simulink model "uncertainities"  (R2021a)
settings: Solver=VariableStepAuto  StartTime=0.0  StopTime=10.0  RelTol=1e-3
settings Model: Creator=jessilbijou  LastModifiedBy=jessilbijou

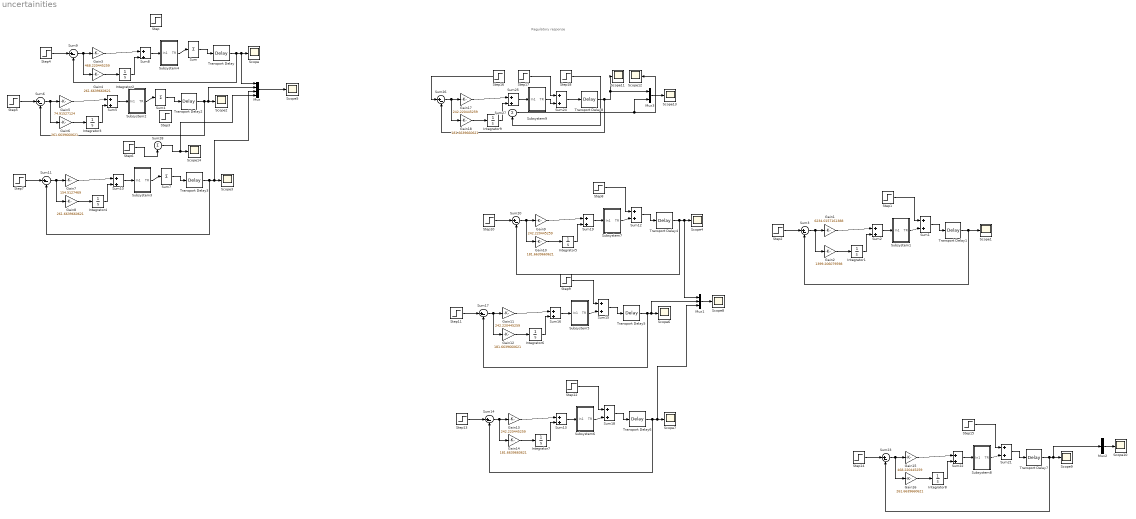
== system uncertainities ==
  note: Regulatory response
  Gain1 : Gain  Gain=6234.0157161388
  Gain{10,12,14,18} (4 alike) : Gain  Gain=181.6639660621
  Gain{9,11,13,17} (4 alike) : Gain  Gain=242.220445259
  Gain15 : Gain  Gain=468.220445259
  Gain{4,6,8,16} (4 alike) : Gain  Gain=261.6639660621
  Gain2 : Gain  Gain=1399.206079598
  Gain3 : Gain  Gain=468.220445259
  Gain5 : Gain  Gain=74.91527124
  Gain7 : Gain  Gain=154.5127469
  Integrator{1..9} (9 alike) : Integrator
  Mux : Mux
  Mux1 : Mux  Inputs=3
  Mux2 : Mux  Inputs=3
  Mux3 : Mux  Inputs=2
  Scope{,1..14} (15 alike) : Scope
  Step{,3,8..9,12} (5 alike) : Step  Time=400  After=-0.2  SampleTime=0
  Step1 : Step  Time=400  After=-0.4  SampleTime=0
  Step{10..11,13..14,18} (5 alike) : Step  Time=0  Before=415  After=418  SampleTime=0
  Step15 : Step  SampleTime=0
  Step16 : Step  Time=80  Before=415  After=418  SampleTime=0
  Step17 : Step  Time=400  After=0.2  SampleTime=0
  Step2 : Step  Time=10  Before=415  After=418  SampleTime=0
  Step{4..7} (4 alike) : Step  Time=70  Before=415  After=418  SampleTime=0
  Subsystem1 : Subsystem
  Subsystem2 : Subsystem
  Subsystem3 : Subsystem
  Subsystem4 : Subsystem
  Subsystem5 : Subsystem
  Subsystem6 : Subsystem
  Subsystem7 : Subsystem
  Subsystem8 : Subsystem
  Subsystem9 : Subsystem
  Sum{,4,7,27..28} (5 alike) : Sum  Inputs=|+
  Sum{1..2,5,8,10,12..13,15..16,18..19,21..22,24..25} (15 alike) : Sum  Inputs=|++
  Sum{3,6,9,11,14,17,20,23,26} (9 alike) : Sum  Inputs=|+-
  Transport Delay{,1..8} (9 alike) : TransportDelay  DelayTime=0
  wires:
  Gain8/1 -> Integrator4/1
  Sum8/1 -> Subsystem4/1(In1)
  Integrator3/1 -> Sum5/2
  Subsystem3/1(TR) -> Sum7/1
  Mux/1 -> Scope5/1
  Step5/1 -> Sum6/1
  Sum/1 -> Transport Delay/1
  Sum4/1 -> Transport Delay2/1
  Step7/1 -> Sum11/1
  Sum10/1 -> Subsystem3/1(In1)
  Gain4/1 -> Integrator2/1
  Transport Delay2/1 -> Sum6/2, Mux/2, Scope2/1
  Gain6/1 -> Integrator3/1
  Sum6/1 -> Gain6/1, Gain5/1
  Integrator2/1 -> Sum8/2
  Sum7/1 -> Transport Delay3/1
  Sum9/1 -> Gain4/1, Gain3/1
  Step4/1 -> Sum9/1
  Integrator4/1 -> Sum10/2
  Gain7/1 -> Sum10/1
  Transport Delay/1 -> Sum9/2, Mux/1, Scope/1
  Subsystem4/1(TR) -> Sum/1
  Sum5/1 -> Subsystem2/1(In1)
  Gain3/1 -> Sum8/1
  Subsystem2/1(TR) -> Sum4/1
  Sum11/1 -> Gain8/1, Gain7/1
  Gain5/1 -> Sum5/1
  Transport Delay3/1 -> Sum11/2, Mux/3, Scope3/1
  Step6/1 -> Sum28/1
  Sum28/1 -> Mux/4, Scope14/1
  Step17/1 -> Sum24/1
  Mux3/1 -> Scope13/1
  Sum26/1 -> Gain18/1, Gain17/1
  Step18/1 -> Sum27/1
  Transport Delay8/1 -> Sum26/2, Mux3/1, Scope11/1
  Sum24/1 -> Transport Delay8/1
  Integrator9/1 -> Sum25/2
  Gain17/1 -> Sum25/1
  Subsystem9/1(TR) -> Sum24/2
  Sum25/1 -> Subsystem9/1(In1)
  Sum27/1 -> Mux3/2, Scope12/1
  Gain18/1 -> Integrator9/1
  Step16/1 -> Sum26/1
  Sum3/1 -> Gain2/1, Gain1/1
  Gain1/1 -> Sum2/1
  Transport Delay7/1 -> Sum23/2, Mux2/2, Scope9/1
  Sum2/1 -> Subsystem1/1(In1)
  Subsystem6/1(TR) -> Sum18/2
  Subsystem1/1(TR) -> Sum1/2
  Step10/1 -> Sum20/1
  Subsystem7/1(TR) -> Sum12/2
  Sum16/1 -> Subsystem5/1(In1)
  Gain10/1 -> Integrator5/1
  Gain15/1 -> Sum22/1
  Sum1/1 -> Transport Delay1/1
  Integrator5/1 -> Sum19/2
  Step9/1 -> Sum15/1
  Step1/1 -> Sum1/1
  Subsystem5/1(TR) -> Sum15/2
  Transport Delay5/1 -> Sum17/2, Mux1/2, Scope6/1
  Step14/1 -> Sum23/1
  Sum17/1 -> Gain12/1, Gain11/1
  Sum13/1 -> Subsystem6/1(In1)
  Integrator1/1 -> Sum2/2
  Sum15/1 -> Transport Delay5/1
  Gain9/1 -> Sum19/1
  Transport Delay1/1 -> Sum3/2, Scope1/1
  Integrator6/1 -> Sum16/2
  Step12/1 -> Sum18/1
  Transport Delay6/1 -> Sum14/2, Mux1/3, Scope7/1
  Step11/1 -> Sum17/1
  Integrator7/1 -> Sum13/2
  Gain13/1 -> Sum13/1
  Sum19/1 -> Subsystem7/1(In1)
  Step15/1 -> Sum21/1
  Sum21/1 -> Transport Delay7/1
  Gain16/1 -> Integrator8/1
  Sum14/1 -> Gain14/1, Gain13/1
  Gain11/1 -> Sum16/1
  Sum22/1 -> Subsystem8/1(In1)
  Transport Delay4/1 -> Sum20/2, Mux1/1, Scope4/1
  Step8/1 -> Sum12/1
  Gain2/1 -> Integrator1/1
  Step13/1 -> Sum14/1
  Sum18/1 -> Transport Delay6/1
  Sum12/1 -> Transport Delay4/1
  Sum23/1 -> Gain16/1, Gain15/1
  Subsystem8/1(TR) -> Sum21/2
  Gain14/1 -> Integrator7/1
  Integrator8/1 -> Sum22/2
  Gain12/1 -> Integrator6/1
  Step2/1 -> Sum3/1
  Mux2/1 -> Scope10/1
  Mux1/1 -> Scope8/1
  Sum20/1 -> Gain10/1, Gain9/1

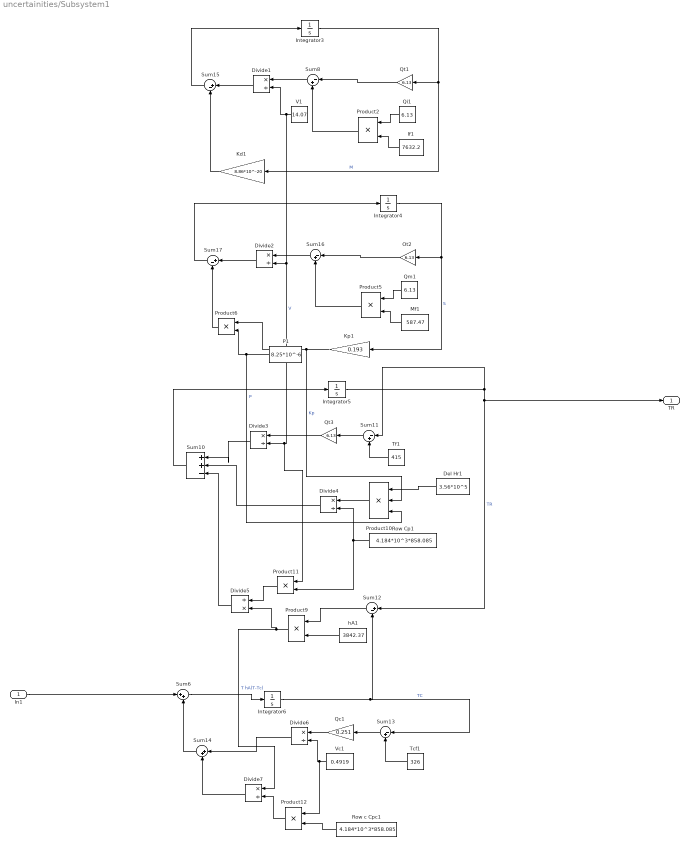
== system uncertainities/Subsystem1 ==
  In1 : Inport
  Del Hr1 : Constant  Value=3.56*10^5
  Divide{1..4,6..7} (6 alike) : Product  Inputs=*/
  Divide5 : Product  Inputs=/*
  If1 : Constant  Value=7632.2
  Integrator3 : Integrator  InitialCondition=7632.2
  Integrator4 : Integrator  InitialCondition=587.47
  Integrator5 : Integrator  InitialCondition=415
  Integrator6 : Integrator  InitialCondition=326
  Kd1 : Gain  Gain=8.86*10^-20
  Kp1 : Gain  Gain=0.193
  Mf1 : Constant  Value=587.47
  Ot2 : Gain  Gain=6.13
  P1 : Constant  Value=8.25*10^-6
  Product10 : Product  Inputs=3
  Product{2,5..6,9,11..12} (6 alike) : Product
  Qc1 : Gain  Gain=0.251
  Qi1 : Constant  Value=6.13
  Qm1 : Constant  Value=6.13
  Qt1 : Gain  Gain=6.13
  Qt3 : Gain  Gain=6.13
  Row Cp1 : Constant  Value=4.184*10^3*858.085
  Row c Cpc1 : Constant  Value=4.184*10^3*858.085
  Sum10 : Sum  Inputs=|++-
  Sum{8,11,13,16} (4 alike) : Sum  Inputs=|-+
  Sum12 : Sum  Inputs=|+-
  Sum14 : Sum  Inputs=|++
  Sum15 : Sum  Inputs=|+-
  Sum17 : Sum  Inputs=|+-
  Sum6 : Sum  Inputs=|++
  Tcf1 : Constant  Value=326
  Tf1 : Constant  Value=415
  V1 : Constant  Value=14.07
  Vc1 : Constant  Value=0.4919
  hA1 : Constant  Value=3842.37
  TR : Outport
  wires:
  Qm1/1 -> Product5/1
  Sum12/1 -> Product9/1
  Sum10/1 -> Integrator5/1
  Integrator5/1 -> TR/1, Sum12/1, Sum11/1  "TR"
  Ot2/1 -> Sum16/1
  Product11/1 -> Divide5/1
  Divide4/1 -> Sum10/2
  Sum16/1 -> Divide2/1
  Del Hr1/1 -> Product10/1
  Qi1/1 -> Product2/1
  Divide5/1 -> Sum10/3
  hA1/1 -> Product9/2
  Row c Cpc1/1 -> Product12/2
  Product10/1 -> Divide4/1
  Kd1/1 -> Sum15/2
  If1/1 -> Product2/2
  Divide3/1 -> Sum10/1
  Product6/1 -> Sum17/2
  Mf1/1 -> Product5/2
  Sum17/1 -> Integrator4/1
  Qt1/1 -> Sum8/1
  Kp1/1 -> Product6/1, Product10/2  "Kp"
  Tcf1/1 -> Sum13/2
  Integrator3/1 -> Kd1/1, Qt1/1  "M"
  Product9/1 -> Divide5/2, Divide7/1  "T hA(T-Tc)"
  Sum15/1 -> Integrator3/1
  Row Cp1/1 -> Product11/2, Divide4/2
  Sum11/1 -> Qt3/1
  Divide1/1 -> Sum15/1
  Product5/1 -> Sum16/2
  P1/1 -> Product6/2, Product10/3  "P"
  Vc1/1 -> Product12/1, Divide6/2
  Product2/1 -> Sum8/2
  V1/1 -> Product11/1, Divide3/2, Divide2/2, Divide1/2  "V"
  Sum8/1 -> Divide1/1
  Integrator4/1 -> Kp1/1, Ot2/1  "S"
  Divide6/1 -> Sum14/1
  Divide2/1 -> Sum17/1
  Divide7/1 -> Sum14/2
  Tf1/1 -> Sum11/2
  Qc1/1 -> Divide6/1
  Sum13/1 -> Qc1/1
  Product12/1 -> Divide7/2
  Integrator6/1 -> Sum13/1, Sum12/2  "TC"
  Qt3/1 -> Divide3/1
  Sum14/1 -> Sum6/2
  In1/1 -> Sum6/1
  Sum6/1 -> Integrator6/1

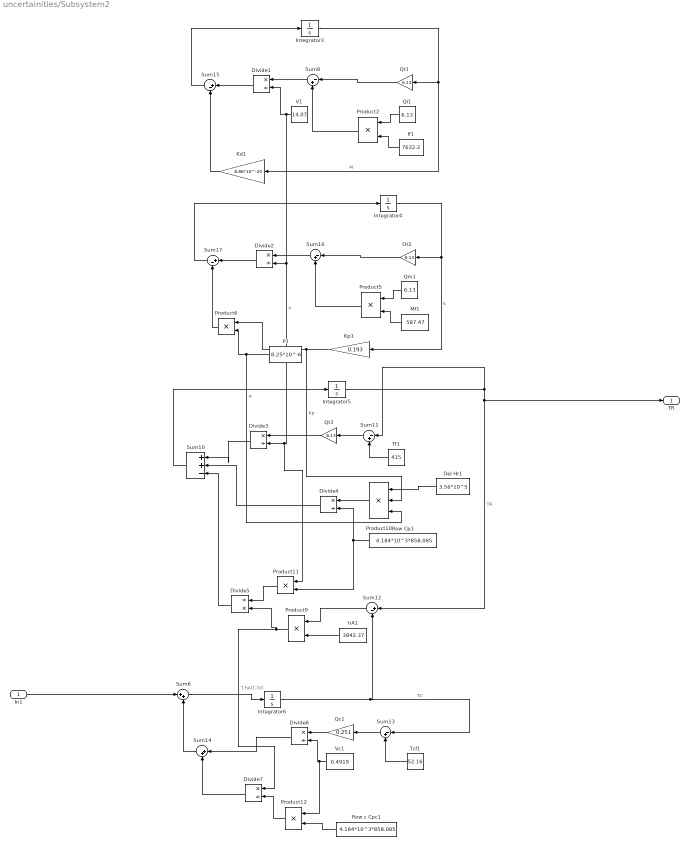
== system uncertainities/Subsystem2 ==
  In1 : Inport
  Del Hr1 : Constant  Value=3.56*10^5
  Divide{1..4,6..7} (6 alike) : Product  Inputs=*/
  Divide5 : Product  Inputs=/*
  If1 : Constant  Value=7632.2
  Integrator3 : Integrator  InitialCondition=7632.2
  Integrator4 : Integrator  InitialCondition=587.47
  Integrator5 : Integrator  InitialCondition=415
  Integrator6 : Integrator  InitialCondition=326
  Kd1 : Gain  Gain=8.86*10^-20
  Kp1 : Gain  Gain=0.193
  Mf1 : Constant  Value=587.47
  Ot2 : Gain  Gain=6.13
  P1 : Constant  Value=8.25*10^-6
  Product10 : Product  Inputs=3
  Product{2,5..6,9,11..12} (6 alike) : Product
  Qc1 : Gain  Gain=0.251
  Qi1 : Constant  Value=6.13
  Qm1 : Constant  Value=6.13
  Qt1 : Gain  Gain=6.13
  Qt3 : Gain  Gain=6.13
  Row Cp1 : Constant  Value=4.184*10^3*858.085
  Row c Cpc1 : Constant  Value=4.184*10^3*858.085
  Sum10 : Sum  Inputs=|++-
  Sum{8,11,13,16} (4 alike) : Sum  Inputs=|-+
  Sum12 : Sum  Inputs=|+-
  Sum14 : Sum  Inputs=|++
  Sum15 : Sum  Inputs=|+-
  Sum17 : Sum  Inputs=|+-
  Sum6 : Sum  Inputs=|++
  Tcf1 : Constant  Value=52.16
  Tf1 : Constant  Value=415
  V1 : Constant  Value=14.07
  Vc1 : Constant  Value=0.4919
  hA1 : Constant  Value=3842.37
  TR : Outport
  wires:
  Qm1/1 -> Product5/1
  Sum12/1 -> Product9/1
  Sum10/1 -> Integrator5/1
  Integrator5/1 -> TR/1, Sum12/1, Sum11/1  "TR"
  Ot2/1 -> Sum16/1
  Product11/1 -> Divide5/1
  Divide4/1 -> Sum10/2
  Sum16/1 -> Divide2/1
  Del Hr1/1 -> Product10/1
  Qi1/1 -> Product2/1
  Divide5/1 -> Sum10/3
  hA1/1 -> Product9/2
  Row c Cpc1/1 -> Product12/2
  Product10/1 -> Divide4/1
  Kd1/1 -> Sum15/2
  If1/1 -> Product2/2
  Divide3/1 -> Sum10/1
  Product6/1 -> Sum17/2
  Mf1/1 -> Product5/2
  Sum17/1 -> Integrator4/1
  Qt1/1 -> Sum8/1
  Kp1/1 -> Product6/1, Product10/2  "Kp"
  Tcf1/1 -> Sum13/2
  Integrator3/1 -> Kd1/1, Qt1/1  "M"
  Product9/1 -> Divide5/2, Divide7/1  "T hA(T-Tc)"
  Sum15/1 -> Integrator3/1
  Row Cp1/1 -> Product11/2, Divide4/2
  Sum11/1 -> Qt3/1
  Divide1/1 -> Sum15/1
  Product5/1 -> Sum16/2
  P1/1 -> Product6/2, Product10/3  "P"
  Vc1/1 -> Product12/1, Divide6/2
  Product2/1 -> Sum8/2
  V1/1 -> Product11/1, Divide3/2, Divide2/2, Divide1/2  "V"
  Sum8/1 -> Divide1/1
  Integrator4/1 -> Kp1/1, Ot2/1  "S"
  Divide6/1 -> Sum14/1
  Divide2/1 -> Sum17/1
  Divide7/1 -> Sum14/2
  Tf1/1 -> Sum11/2
  Qc1/1 -> Divide6/1
  Sum13/1 -> Qc1/1
  Product12/1 -> Divide7/2
  Integrator6/1 -> Sum13/1, Sum12/2  "TC"
  Qt3/1 -> Divide3/1
  Sum14/1 -> Sum6/2
  In1/1 -> Sum6/1
  Sum6/1 -> Integrator6/1

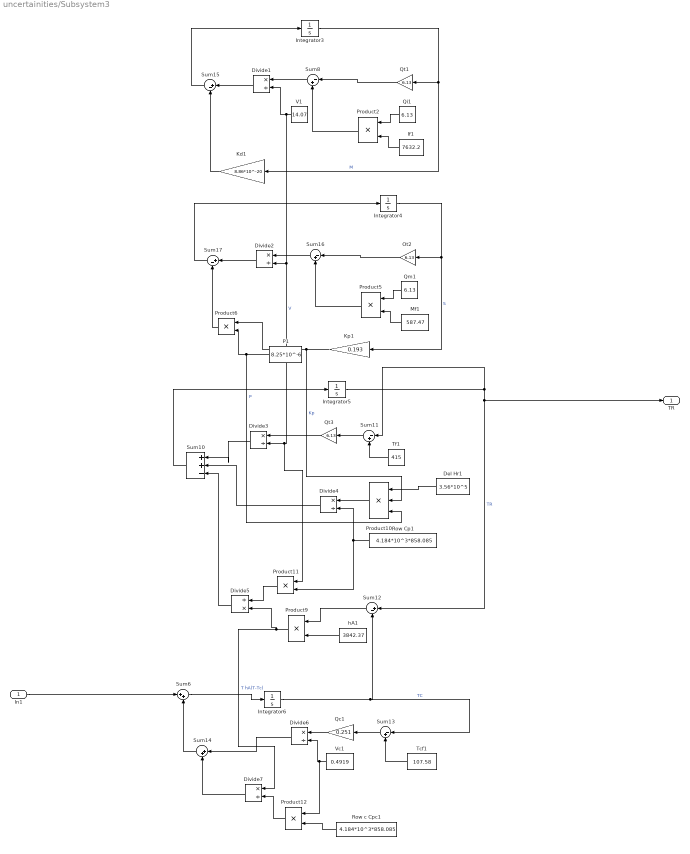
== system uncertainities/Subsystem3 ==
  In1 : Inport
  Del Hr1 : Constant  Value=3.56*10^5
  Divide{1..4,6..7} (6 alike) : Product  Inputs=*/
  Divide5 : Product  Inputs=/*
  If1 : Constant  Value=7632.2
  Integrator3 : Integrator  InitialCondition=7632.2
  Integrator4 : Integrator  InitialCondition=587.47
  Integrator5 : Integrator  InitialCondition=415
  Integrator6 : Integrator  InitialCondition=326
  Kd1 : Gain  Gain=8.86*10^-20
  Kp1 : Gain  Gain=0.193
  Mf1 : Constant  Value=587.47
  Ot2 : Gain  Gain=6.13
  P1 : Constant  Value=8.25*10^-6
  Product10 : Product  Inputs=3
  Product{2,5..6,9,11..12} (6 alike) : Product
  Qc1 : Gain  Gain=0.251
  Qi1 : Constant  Value=6.13
  Qm1 : Constant  Value=6.13
  Qt1 : Gain  Gain=6.13
  Qt3 : Gain  Gain=6.13
  Row Cp1 : Constant  Value=4.184*10^3*858.085
  Row c Cpc1 : Constant  Value=4.184*10^3*858.085
  Sum10 : Sum  Inputs=|++-
  Sum{8,11,13,16} (4 alike) : Sum  Inputs=|-+
  Sum12 : Sum  Inputs=|+-
  Sum14 : Sum  Inputs=|++
  Sum15 : Sum  Inputs=|+-
  Sum17 : Sum  Inputs=|+-
  Sum6 : Sum  Inputs=|++
  Tcf1 : Constant  Value=107.58
  Tf1 : Constant  Value=415
  V1 : Constant  Value=14.07
  Vc1 : Constant  Value=0.4919
  hA1 : Constant  Value=3842.37
  TR : Outport
  wires:
  Qm1/1 -> Product5/1
  Sum12/1 -> Product9/1
  Sum10/1 -> Integrator5/1
  Integrator5/1 -> TR/1, Sum12/1, Sum11/1  "TR"
  Ot2/1 -> Sum16/1
  Product11/1 -> Divide5/1
  Divide4/1 -> Sum10/2
  Sum16/1 -> Divide2/1
  Del Hr1/1 -> Product10/1
  Qi1/1 -> Product2/1
  Divide5/1 -> Sum10/3
  hA1/1 -> Product9/2
  Row c Cpc1/1 -> Product12/2
  Product10/1 -> Divide4/1
  Kd1/1 -> Sum15/2
  If1/1 -> Product2/2
  Divide3/1 -> Sum10/1
  Product6/1 -> Sum17/2
  Mf1/1 -> Product5/2
  Sum17/1 -> Integrator4/1
  Qt1/1 -> Sum8/1
  Kp1/1 -> Product6/1, Product10/2  "Kp"
  Tcf1/1 -> Sum13/2
  Integrator3/1 -> Kd1/1, Qt1/1  "M"
  Product9/1 -> Divide5/2, Divide7/1  "T hA(T-Tc)"
  Sum15/1 -> Integrator3/1
  Row Cp1/1 -> Product11/2, Divide4/2
  Sum11/1 -> Qt3/1
  Divide1/1 -> Sum15/1
  Product5/1 -> Sum16/2
  P1/1 -> Product6/2, Product10/3  "P"
  Vc1/1 -> Product12/1, Divide6/2
  Product2/1 -> Sum8/2
  V1/1 -> Product11/1, Divide3/2, Divide2/2, Divide1/2  "V"
  Sum8/1 -> Divide1/1
  Integrator4/1 -> Kp1/1, Ot2/1  "S"
  Divide6/1 -> Sum14/1
  Divide2/1 -> Sum17/1
  Divide7/1 -> Sum14/2
  Tf1/1 -> Sum11/2
  Qc1/1 -> Divide6/1
  Sum13/1 -> Qc1/1
  Product12/1 -> Divide7/2
  Integrator6/1 -> Sum13/1, Sum12/2  "TC"
  Qt3/1 -> Divide3/1
  Sum14/1 -> Sum6/2
  In1/1 -> Sum6/1
  Sum6/1 -> Integrator6/1

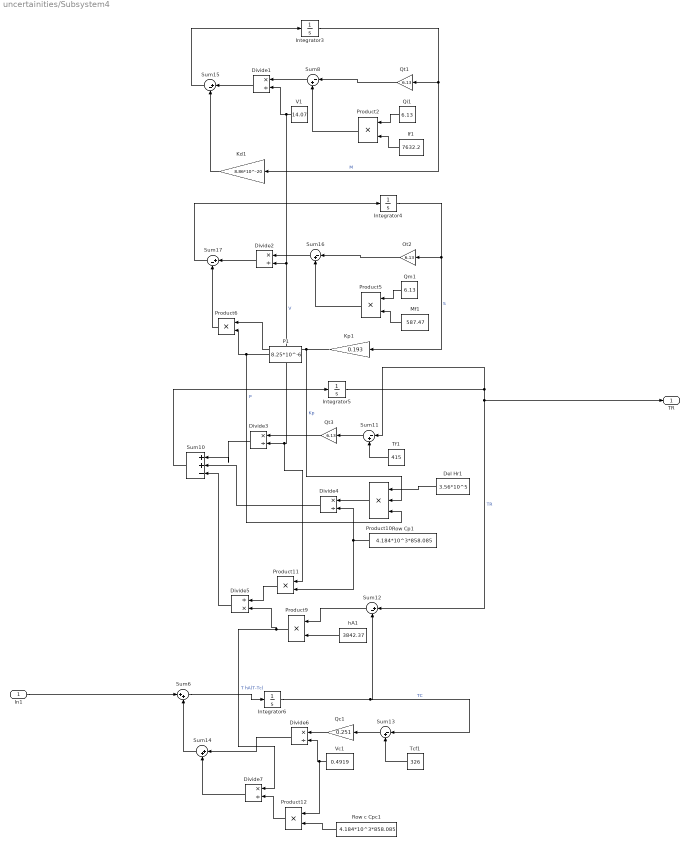
== system uncertainities/Subsystem4 ==
  In1 : Inport
  Del Hr1 : Constant  Value=3.56*10^5
  Divide{1..4,6..7} (6 alike) : Product  Inputs=*/
  Divide5 : Product  Inputs=/*
  If1 : Constant  Value=7632.2
  Integrator3 : Integrator  InitialCondition=7632.2
  Integrator4 : Integrator  InitialCondition=587.47
  Integrator5 : Integrator  InitialCondition=415
  Integrator6 : Integrator  InitialCondition=326
  Kd1 : Gain  Gain=8.86*10^-20
  Kp1 : Gain  Gain=0.193
  Mf1 : Constant  Value=587.47
  Ot2 : Gain  Gain=6.13
  P1 : Constant  Value=8.25*10^-6
  Product10 : Product  Inputs=3
  Product{2,5..6,9,11..12} (6 alike) : Product
  Qc1 : Gain  Gain=0.251
  Qi1 : Constant  Value=6.13
  Qm1 : Constant  Value=6.13
  Qt1 : Gain  Gain=6.13
  Qt3 : Gain  Gain=6.13
  Row Cp1 : Constant  Value=4.184*10^3*858.085
  Row c Cpc1 : Constant  Value=4.184*10^3*858.085
  Sum10 : Sum  Inputs=|++-
  Sum{8,11,13,16} (4 alike) : Sum  Inputs=|-+
  Sum12 : Sum  Inputs=|+-
  Sum14 : Sum  Inputs=|++
  Sum15 : Sum  Inputs=|+-
  Sum17 : Sum  Inputs=|+-
  Sum6 : Sum  Inputs=|++
  Tcf1 : Constant  Value=326
  Tf1 : Constant  Value=415
  V1 : Constant  Value=14.07
  Vc1 : Constant  Value=0.4919
  hA1 : Constant  Value=3842.37
  TR : Outport
  wires:
  Qm1/1 -> Product5/1
  Sum12/1 -> Product9/1
  Sum10/1 -> Integrator5/1
  Integrator5/1 -> TR/1, Sum12/1, Sum11/1  "TR"
  Ot2/1 -> Sum16/1
  Product11/1 -> Divide5/1
  Divide4/1 -> Sum10/2
  Sum16/1 -> Divide2/1
  Del Hr1/1 -> Product10/1
  Qi1/1 -> Product2/1
  Divide5/1 -> Sum10/3
  hA1/1 -> Product9/2
  Row c Cpc1/1 -> Product12/2
  Product10/1 -> Divide4/1
  Kd1/1 -> Sum15/2
  If1/1 -> Product2/2
  Divide3/1 -> Sum10/1
  Product6/1 -> Sum17/2
  Mf1/1 -> Product5/2
  Sum17/1 -> Integrator4/1
  Qt1/1 -> Sum8/1
  Kp1/1 -> Product6/1, Product10/2  "Kp"
  Tcf1/1 -> Sum13/2
  Integrator3/1 -> Kd1/1, Qt1/1  "M"
  Product9/1 -> Divide5/2, Divide7/1  "T hA(T-Tc)"
  Sum15/1 -> Integrator3/1
  Row Cp1/1 -> Product11/2, Divide4/2
  Sum11/1 -> Qt3/1
  Divide1/1 -> Sum15/1
  Product5/1 -> Sum16/2
  P1/1 -> Product6/2, Product10/3  "P"
  Vc1/1 -> Product12/1, Divide6/2
  Product2/1 -> Sum8/2
  V1/1 -> Product11/1, Divide3/2, Divide2/2, Divide1/2  "V"
  Sum8/1 -> Divide1/1
  Integrator4/1 -> Kp1/1, Ot2/1  "S"
  Divide6/1 -> Sum14/1
  Divide2/1 -> Sum17/1
  Divide7/1 -> Sum14/2
  Tf1/1 -> Sum11/2
  Qc1/1 -> Divide6/1
  Sum13/1 -> Qc1/1
  Product12/1 -> Divide7/2
  Integrator6/1 -> Sum13/1, Sum12/2  "TC"
  Qt3/1 -> Divide3/1
  Sum14/1 -> Sum6/2
  In1/1 -> Sum6/1
  Sum6/1 -> Integrator6/1

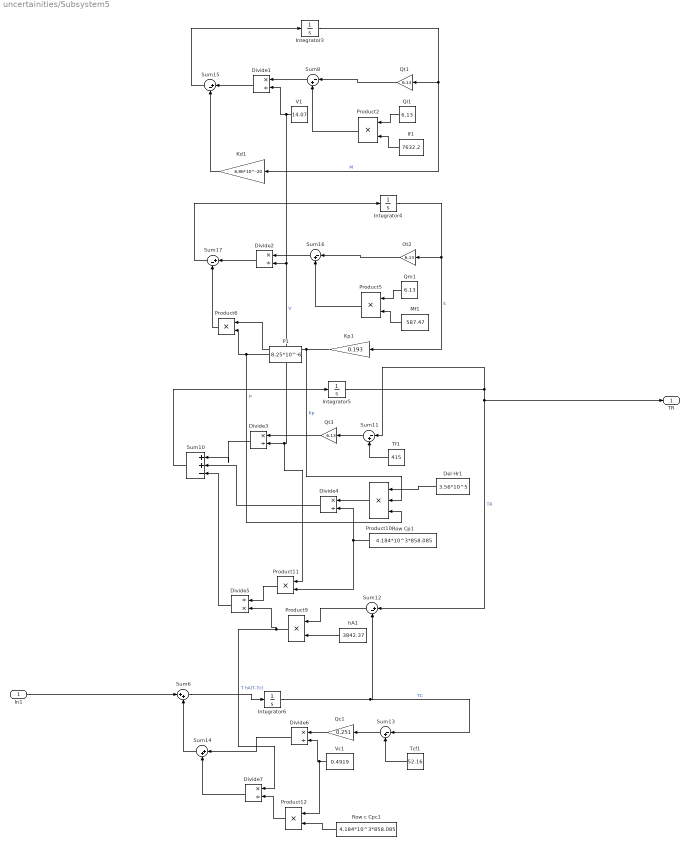
== system uncertainities/Subsystem5 ==
  In1 : Inport
  Del Hr1 : Constant  Value=3.56*10^5
  Divide{1..4,6..7} (6 alike) : Product  Inputs=*/
  Divide5 : Product  Inputs=/*
  If1 : Constant  Value=7632.2
  Integrator3 : Integrator  InitialCondition=7632.2
  Integrator4 : Integrator  InitialCondition=587.47
  Integrator5 : Integrator  InitialCondition=415
  Integrator6 : Integrator  InitialCondition=326
  Kd1 : Gain  Gain=8.86*10^-20
  Kp1 : Gain  Gain=0.193
  Mf1 : Constant  Value=587.47
  Ot2 : Gain  Gain=6.13
  P1 : Constant  Value=8.25*10^-6
  Product10 : Product  Inputs=3
  Product{2,5..6,9,11..12} (6 alike) : Product
  Qc1 : Gain  Gain=0.251
  Qi1 : Constant  Value=6.13
  Qm1 : Constant  Value=6.13
  Qt1 : Gain  Gain=6.13
  Qt3 : Gain  Gain=6.13
  Row Cp1 : Constant  Value=4.184*10^3*858.085
  Row c Cpc1 : Constant  Value=4.184*10^3*858.085
  Sum10 : Sum  Inputs=|++-
  Sum{8,11,13,16} (4 alike) : Sum  Inputs=|-+
  Sum12 : Sum  Inputs=|+-
  Sum14 : Sum  Inputs=|++
  Sum15 : Sum  Inputs=|+-
  Sum17 : Sum  Inputs=|+-
  Sum6 : Sum  Inputs=|++
  Tcf1 : Constant  Value=52.16
  Tf1 : Constant  Value=415
  V1 : Constant  Value=14.07
  Vc1 : Constant  Value=0.4919
  hA1 : Constant  Value=3842.37
  TR : Outport
  wires:
  Qm1/1 -> Product5/1
  Sum12/1 -> Product9/1
  Sum10/1 -> Integrator5/1
  Integrator5/1 -> TR/1, Sum12/1, Sum11/1  "TR"
  Ot2/1 -> Sum16/1
  Product11/1 -> Divide5/1
  Divide4/1 -> Sum10/2
  Sum16/1 -> Divide2/1
  Del Hr1/1 -> Product10/1
  Qi1/1 -> Product2/1
  Divide5/1 -> Sum10/3
  hA1/1 -> Product9/2
  Row c Cpc1/1 -> Product12/2
  Product10/1 -> Divide4/1
  Kd1/1 -> Sum15/2
  If1/1 -> Product2/2
  Divide3/1 -> Sum10/1
  Product6/1 -> Sum17/2
  Mf1/1 -> Product5/2
  Sum17/1 -> Integrator4/1
  Qt1/1 -> Sum8/1
  Kp1/1 -> Product6/1, Product10/2  "Kp"
  Tcf1/1 -> Sum13/2
  Integrator3/1 -> Kd1/1, Qt1/1  "M"
  Product9/1 -> Divide5/2, Divide7/1  "T hA(T-Tc)"
  Sum15/1 -> Integrator3/1
  Row Cp1/1 -> Product11/2, Divide4/2
  Sum11/1 -> Qt3/1
  Divide1/1 -> Sum15/1
  Product5/1 -> Sum16/2
  P1/1 -> Product6/2, Product10/3  "P"
  Vc1/1 -> Product12/1, Divide6/2
  Product2/1 -> Sum8/2
  V1/1 -> Product11/1, Divide3/2, Divide2/2, Divide1/2  "V"
  Sum8/1 -> Divide1/1
  Integrator4/1 -> Kp1/1, Ot2/1  "S"
  Divide6/1 -> Sum14/1
  Divide2/1 -> Sum17/1
  Divide7/1 -> Sum14/2
  Tf1/1 -> Sum11/2
  Qc1/1 -> Divide6/1
  Sum13/1 -> Qc1/1
  Product12/1 -> Divide7/2
  Integrator6/1 -> Sum13/1, Sum12/2  "TC"
  Qt3/1 -> Divide3/1
  Sum14/1 -> Sum6/2
  In1/1 -> Sum6/1
  Sum6/1 -> Integrator6/1

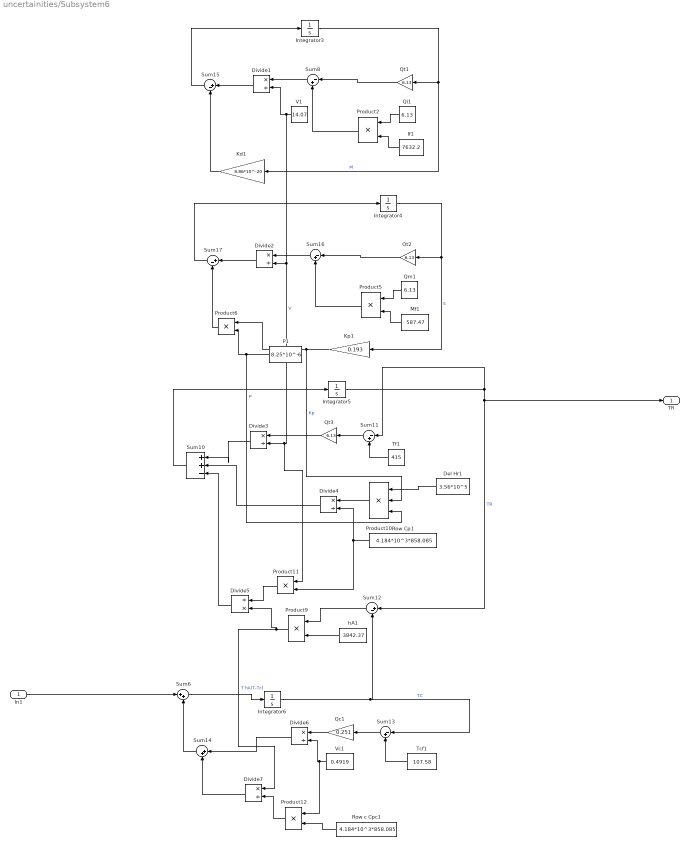
== system uncertainities/Subsystem6 ==
  In1 : Inport
  Del Hr1 : Constant  Value=3.56*10^5
  Divide{1..4,6..7} (6 alike) : Product  Inputs=*/
  Divide5 : Product  Inputs=/*
  If1 : Constant  Value=7632.2
  Integrator3 : Integrator  InitialCondition=7632.2
  Integrator4 : Integrator  InitialCondition=587.47
  Integrator5 : Integrator  InitialCondition=415
  Integrator6 : Integrator  InitialCondition=326
  Kd1 : Gain  Gain=8.86*10^-20
  Kp1 : Gain  Gain=0.193
  Mf1 : Constant  Value=587.47
  Ot2 : Gain  Gain=6.13
  P1 : Constant  Value=8.25*10^-6
  Product10 : Product  Inputs=3
  Product{2,5..6,9,11..12} (6 alike) : Product
  Qc1 : Gain  Gain=0.251
  Qi1 : Constant  Value=6.13
  Qm1 : Constant  Value=6.13
  Qt1 : Gain  Gain=6.13
  Qt3 : Gain  Gain=6.13
  Row Cp1 : Constant  Value=4.184*10^3*858.085
  Row c Cpc1 : Constant  Value=4.184*10^3*858.085
  Sum10 : Sum  Inputs=|++-
  Sum{8,11,13,16} (4 alike) : Sum  Inputs=|-+
  Sum12 : Sum  Inputs=|+-
  Sum14 : Sum  Inputs=|++
  Sum15 : Sum  Inputs=|+-
  Sum17 : Sum  Inputs=|+-
  Sum6 : Sum  Inputs=|++
  Tcf1 : Constant  Value=107.58
  Tf1 : Constant  Value=415
  V1 : Constant  Value=14.07
  Vc1 : Constant  Value=0.4919
  hA1 : Constant  Value=3842.37
  TR : Outport
  wires:
  Qm1/1 -> Product5/1
  Sum12/1 -> Product9/1
  Sum10/1 -> Integrator5/1
  Integrator5/1 -> TR/1, Sum12/1, Sum11/1  "TR"
  Ot2/1 -> Sum16/1
  Product11/1 -> Divide5/1
  Divide4/1 -> Sum10/2
  Sum16/1 -> Divide2/1
  Del Hr1/1 -> Product10/1
  Qi1/1 -> Product2/1
  Divide5/1 -> Sum10/3
  hA1/1 -> Product9/2
  Row c Cpc1/1 -> Product12/2
  Product10/1 -> Divide4/1
  Kd1/1 -> Sum15/2
  If1/1 -> Product2/2
  Divide3/1 -> Sum10/1
  Product6/1 -> Sum17/2
  Mf1/1 -> Product5/2
  Sum17/1 -> Integrator4/1
  Qt1/1 -> Sum8/1
  Kp1/1 -> Product6/1, Product10/2  "Kp"
  Tcf1/1 -> Sum13/2
  Integrator3/1 -> Kd1/1, Qt1/1  "M"
  Product9/1 -> Divide5/2, Divide7/1  "T hA(T-Tc)"
  Sum15/1 -> Integrator3/1
  Row Cp1/1 -> Product11/2, Divide4/2
  Sum11/1 -> Qt3/1
  Divide1/1 -> Sum15/1
  Product5/1 -> Sum16/2
  P1/1 -> Product6/2, Product10/3  "P"
  Vc1/1 -> Product12/1, Divide6/2
  Product2/1 -> Sum8/2
  V1/1 -> Product11/1, Divide3/2, Divide2/2, Divide1/2  "V"
  Sum8/1 -> Divide1/1
  Integrator4/1 -> Kp1/1, Ot2/1  "S"
  Divide6/1 -> Sum14/1
  Divide2/1 -> Sum17/1
  Divide7/1 -> Sum14/2
  Tf1/1 -> Sum11/2
  Qc1/1 -> Divide6/1
  Sum13/1 -> Qc1/1
  Product12/1 -> Divide7/2
  Integrator6/1 -> Sum13/1, Sum12/2  "TC"
  Qt3/1 -> Divide3/1
  Sum14/1 -> Sum6/2
  In1/1 -> Sum6/1
  Sum6/1 -> Integrator6/1

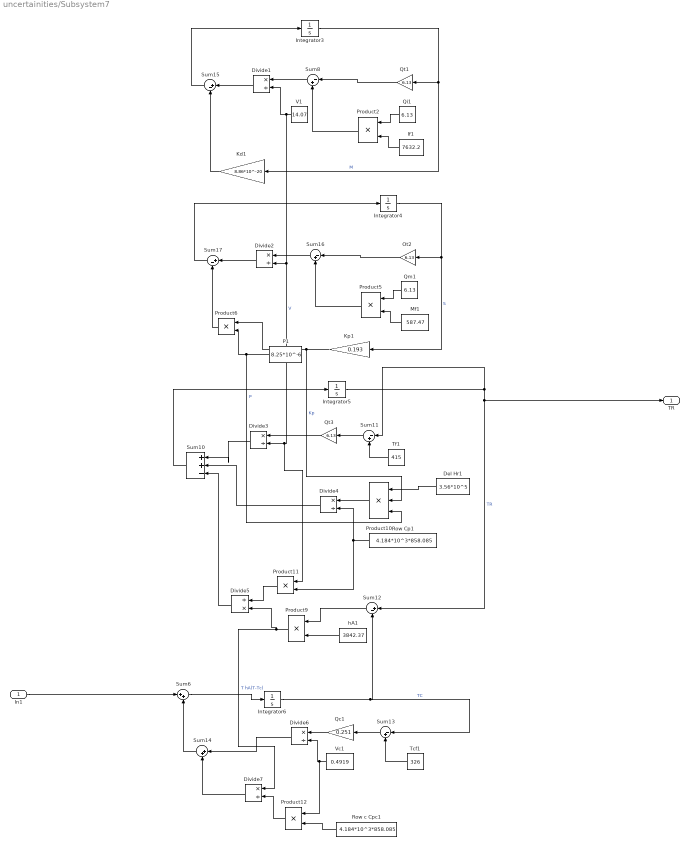
== system uncertainities/Subsystem7 ==
  In1 : Inport
  Del Hr1 : Constant  Value=3.56*10^5
  Divide{1..4,6..7} (6 alike) : Product  Inputs=*/
  Divide5 : Product  Inputs=/*
  If1 : Constant  Value=7632.2
  Integrator3 : Integrator  InitialCondition=7632.2
  Integrator4 : Integrator  InitialCondition=587.47
  Integrator5 : Integrator  InitialCondition=415
  Integrator6 : Integrator  InitialCondition=326
  Kd1 : Gain  Gain=8.86*10^-20
  Kp1 : Gain  Gain=0.193
  Mf1 : Constant  Value=587.47
  Ot2 : Gain  Gain=6.13
  P1 : Constant  Value=8.25*10^-6
  Product10 : Product  Inputs=3
  Product{2,5..6,9,11..12} (6 alike) : Product
  Qc1 : Gain  Gain=0.251
  Qi1 : Constant  Value=6.13
  Qm1 : Constant  Value=6.13
  Qt1 : Gain  Gain=6.13
  Qt3 : Gain  Gain=6.13
  Row Cp1 : Constant  Value=4.184*10^3*858.085
  Row c Cpc1 : Constant  Value=4.184*10^3*858.085
  Sum10 : Sum  Inputs=|++-
  Sum{8,11,13,16} (4 alike) : Sum  Inputs=|-+
  Sum12 : Sum  Inputs=|+-
  Sum14 : Sum  Inputs=|++
  Sum15 : Sum  Inputs=|+-
  Sum17 : Sum  Inputs=|+-
  Sum6 : Sum  Inputs=|++
  Tcf1 : Constant  Value=326
  Tf1 : Constant  Value=415
  V1 : Constant  Value=14.07
  Vc1 : Constant  Value=0.4919
  hA1 : Constant  Value=3842.37
  TR : Outport
  wires:
  Qm1/1 -> Product5/1
  Sum12/1 -> Product9/1
  Sum10/1 -> Integrator5/1
  Integrator5/1 -> TR/1, Sum12/1, Sum11/1  "TR"
  Ot2/1 -> Sum16/1
  Product11/1 -> Divide5/1
  Divide4/1 -> Sum10/2
  Sum16/1 -> Divide2/1
  Del Hr1/1 -> Product10/1
  Qi1/1 -> Product2/1
  Divide5/1 -> Sum10/3
  hA1/1 -> Product9/2
  Row c Cpc1/1 -> Product12/2
  Product10/1 -> Divide4/1
  Kd1/1 -> Sum15/2
  If1/1 -> Product2/2
  Divide3/1 -> Sum10/1
  Product6/1 -> Sum17/2
  Mf1/1 -> Product5/2
  Sum17/1 -> Integrator4/1
  Qt1/1 -> Sum8/1
  Kp1/1 -> Product6/1, Product10/2  "Kp"
  Tcf1/1 -> Sum13/2
  Integrator3/1 -> Kd1/1, Qt1/1  "M"
  Product9/1 -> Divide5/2, Divide7/1  "T hA(T-Tc)"
  Sum15/1 -> Integrator3/1
  Row Cp1/1 -> Product11/2, Divide4/2
  Sum11/1 -> Qt3/1
  Divide1/1 -> Sum15/1
  Product5/1 -> Sum16/2
  P1/1 -> Product6/2, Product10/3  "P"
  Vc1/1 -> Product12/1, Divide6/2
  Product2/1 -> Sum8/2
  V1/1 -> Product11/1, Divide3/2, Divide2/2, Divide1/2  "V"
  Sum8/1 -> Divide1/1
  Integrator4/1 -> Kp1/1, Ot2/1  "S"
  Divide6/1 -> Sum14/1
  Divide2/1 -> Sum17/1
  Divide7/1 -> Sum14/2
  Tf1/1 -> Sum11/2
  Qc1/1 -> Divide6/1
  Sum13/1 -> Qc1/1
  Product12/1 -> Divide7/2
  Integrator6/1 -> Sum13/1, Sum12/2  "TC"
  Qt3/1 -> Divide3/1
  Sum14/1 -> Sum6/2
  In1/1 -> Sum6/1
  Sum6/1 -> Integrator6/1

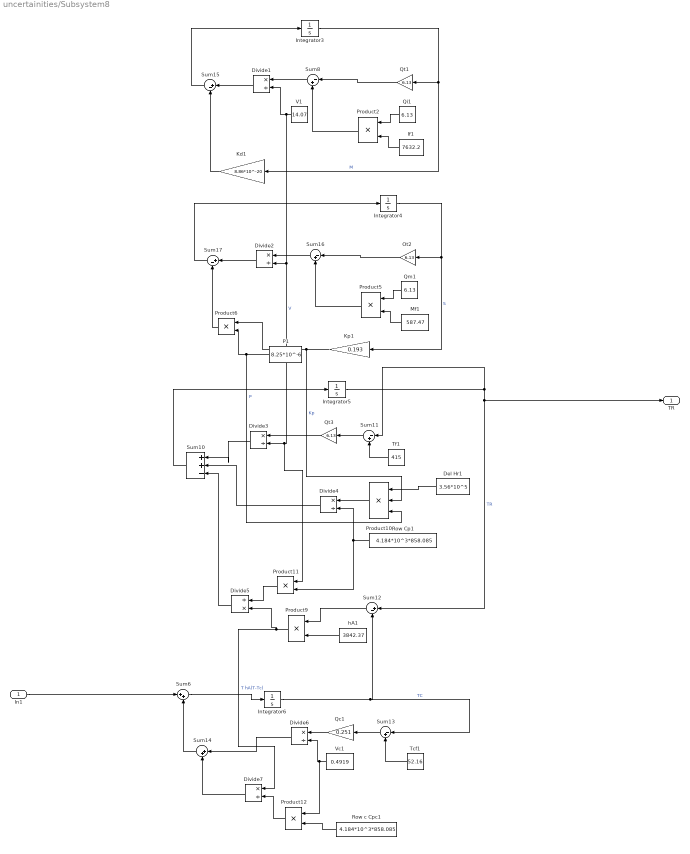
== system uncertainities/Subsystem8 ==
  In1 : Inport
  Del Hr1 : Constant  Value=3.56*10^5
  Divide{1..4,6..7} (6 alike) : Product  Inputs=*/
  Divide5 : Product  Inputs=/*
  If1 : Constant  Value=7632.2
  Integrator3 : Integrator  InitialCondition=7632.2
  Integrator4 : Integrator  InitialCondition=587.47
  Integrator5 : Integrator  InitialCondition=415
  Integrator6 : Integrator  InitialCondition=326
  Kd1 : Gain  Gain=8.86*10^-20
  Kp1 : Gain  Gain=0.193
  Mf1 : Constant  Value=587.47
  Ot2 : Gain  Gain=6.13
  P1 : Constant  Value=8.25*10^-6
  Product10 : Product  Inputs=3
  Product{2,5..6,9,11..12} (6 alike) : Product
  Qc1 : Gain  Gain=0.251
  Qi1 : Constant  Value=6.13
  Qm1 : Constant  Value=6.13
  Qt1 : Gain  Gain=6.13
  Qt3 : Gain  Gain=6.13
  Row Cp1 : Constant  Value=4.184*10^3*858.085
  Row c Cpc1 : Constant  Value=4.184*10^3*858.085
  Sum10 : Sum  Inputs=|++-
  Sum{8,11,13,16} (4 alike) : Sum  Inputs=|-+
  Sum12 : Sum  Inputs=|+-
  Sum14 : Sum  Inputs=|++
  Sum15 : Sum  Inputs=|+-
  Sum17 : Sum  Inputs=|+-
  Sum6 : Sum  Inputs=|++
  Tcf1 : Constant  Value=52.16
  Tf1 : Constant  Value=415
  V1 : Constant  Value=14.07
  Vc1 : Constant  Value=0.4919
  hA1 : Constant  Value=3842.37
  TR : Outport
  wires:
  Qm1/1 -> Product5/1
  Sum12/1 -> Product9/1
  Sum10/1 -> Integrator5/1
  Integrator5/1 -> TR/1, Sum12/1, Sum11/1  "TR"
  Ot2/1 -> Sum16/1
  Product11/1 -> Divide5/1
  Divide4/1 -> Sum10/2
  Sum16/1 -> Divide2/1
  Del Hr1/1 -> Product10/1
  Qi1/1 -> Product2/1
  Divide5/1 -> Sum10/3
  hA1/1 -> Product9/2
  Row c Cpc1/1 -> Product12/2
  Product10/1 -> Divide4/1
  Kd1/1 -> Sum15/2
  If1/1 -> Product2/2
  Divide3/1 -> Sum10/1
  Product6/1 -> Sum17/2
  Mf1/1 -> Product5/2
  Sum17/1 -> Integrator4/1
  Qt1/1 -> Sum8/1
  Kp1/1 -> Product6/1, Product10/2  "Kp"
  Tcf1/1 -> Sum13/2
  Integrator3/1 -> Kd1/1, Qt1/1  "M"
  Product9/1 -> Divide5/2, Divide7/1  "T hA(T-Tc)"
  Sum15/1 -> Integrator3/1
  Row Cp1/1 -> Product11/2, Divide4/2
  Sum11/1 -> Qt3/1
  Divide1/1 -> Sum15/1
  Product5/1 -> Sum16/2
  P1/1 -> Product6/2, Product10/3  "P"
  Vc1/1 -> Product12/1, Divide6/2
  Product2/1 -> Sum8/2
  V1/1 -> Product11/1, Divide3/2, Divide2/2, Divide1/2  "V"
  Sum8/1 -> Divide1/1
  Integrator4/1 -> Kp1/1, Ot2/1  "S"
  Divide6/1 -> Sum14/1
  Divide2/1 -> Sum17/1
  Divide7/1 -> Sum14/2
  Tf1/1 -> Sum11/2
  Qc1/1 -> Divide6/1
  Sum13/1 -> Qc1/1
  Product12/1 -> Divide7/2
  Integrator6/1 -> Sum13/1, Sum12/2  "TC"
  Qt3/1 -> Divide3/1
  Sum14/1 -> Sum6/2
  In1/1 -> Sum6/1
  Sum6/1 -> Integrator6/1

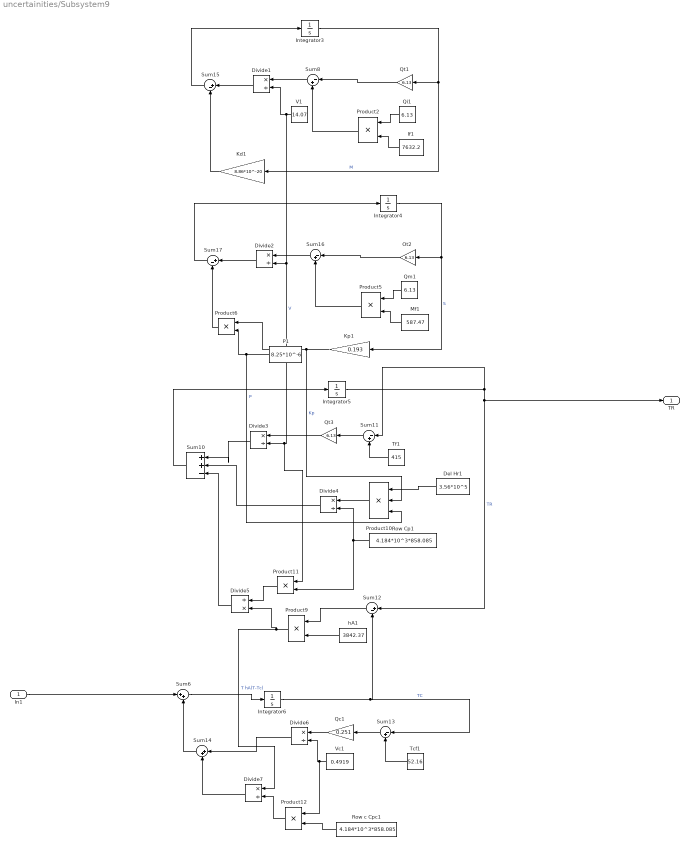
== system uncertainities/Subsystem9 ==
  In1 : Inport
  Del Hr1 : Constant  Value=3.56*10^5
  Divide{1..4,6..7} (6 alike) : Product  Inputs=*/
  Divide5 : Product  Inputs=/*
  If1 : Constant  Value=7632.2
  Integrator3 : Integrator  InitialCondition=7632.2
  Integrator4 : Integrator  InitialCondition=587.47
  Integrator5 : Integrator  InitialCondition=415
  Integrator6 : Integrator  InitialCondition=326
  Kd1 : Gain  Gain=8.86*10^-20
  Kp1 : Gain  Gain=0.193
  Mf1 : Constant  Value=587.47
  Ot2 : Gain  Gain=6.13
  P1 : Constant  Value=8.25*10^-6
  Product10 : Product  Inputs=3
  Product{2,5..6,9,11..12} (6 alike) : Product
  Qc1 : Gain  Gain=0.251
  Qi1 : Constant  Value=6.13
  Qm1 : Constant  Value=6.13
  Qt1 : Gain  Gain=6.13
  Qt3 : Gain  Gain=6.13
  Row Cp1 : Constant  Value=4.184*10^3*858.085
  Row c Cpc1 : Constant  Value=4.184*10^3*858.085
  Sum10 : Sum  Inputs=|++-
  Sum{8,11,13,16} (4 alike) : Sum  Inputs=|-+
  Sum12 : Sum  Inputs=|+-
  Sum14 : Sum  Inputs=|++
  Sum15 : Sum  Inputs=|+-
  Sum17 : Sum  Inputs=|+-
  Sum6 : Sum  Inputs=|++
  Tcf1 : Constant  Value=52.16
  Tf1 : Constant  Value=415
  V1 : Constant  Value=14.07
  Vc1 : Constant  Value=0.4919
  hA1 : Constant  Value=3842.37
  TR : Outport
  wires:
  Qm1/1 -> Product5/1
  Sum12/1 -> Product9/1
  Sum10/1 -> Integrator5/1
  Integrator5/1 -> TR/1, Sum12/1, Sum11/1  "TR"
  Ot2/1 -> Sum16/1
  Product11/1 -> Divide5/1
  Divide4/1 -> Sum10/2
  Sum16/1 -> Divide2/1
  Del Hr1/1 -> Product10/1
  Qi1/1 -> Product2/1
  Divide5/1 -> Sum10/3
  hA1/1 -> Product9/2
  Row c Cpc1/1 -> Product12/2
  Product10/1 -> Divide4/1
  Kd1/1 -> Sum15/2
  If1/1 -> Product2/2
  Divide3/1 -> Sum10/1
  Product6/1 -> Sum17/2
  Mf1/1 -> Product5/2
  Sum17/1 -> Integrator4/1
  Qt1/1 -> Sum8/1
  Kp1/1 -> Product6/1, Product10/2  "Kp"
  Tcf1/1 -> Sum13/2
  Integrator3/1 -> Kd1/1, Qt1/1  "M"
  Product9/1 -> Divide5/2, Divide7/1  "T hA(T-Tc)"
  Sum15/1 -> Integrator3/1
  Row Cp1/1 -> Product11/2, Divide4/2
  Sum11/1 -> Qt3/1
  Divide1/1 -> Sum15/1
  Product5/1 -> Sum16/2
  P1/1 -> Product6/2, Product10/3  "P"
  Vc1/1 -> Product12/1, Divide6/2
  Product2/1 -> Sum8/2
  V1/1 -> Product11/1, Divide3/2, Divide2/2, Divide1/2  "V"
  Sum8/1 -> Divide1/1
  Integrator4/1 -> Kp1/1, Ot2/1  "S"
  Divide6/1 -> Sum14/1
  Divide2/1 -> Sum17/1
  Divide7/1 -> Sum14/2
  Tf1/1 -> Sum11/2
  Qc1/1 -> Divide6/1
  Sum13/1 -> Qc1/1
  Product12/1 -> Divide7/2
  Integrator6/1 -> Sum13/1, Sum12/2  "TC"
  Qt3/1 -> Divide3/1
  Sum14/1 -> Sum6/2
  In1/1 -> Sum6/1
  Sum6/1 -> Integrator6/1
